simulink model "Simulacao_3DANIM"  (R2021a)
settings: Solver=ode4  StartTime=0.0  StopTime=300  FixedStep=0.01  RelTol=1e-3  EnableMultiTasking=on
values from neighbouring files (symbols this model uses):
  Ka = 4.5    [INICIO.m]
  Kdc = 1.1    [INICIO.m]
  Ki = 14.3    [INICIO.m]
  Kr = -0.37    [INICIO.m]
  l_M0 = 80*d2r    (= 1.3962634016)    [INICIO.m]
  l_T0 = -2.5*d2r    (= -0.0436332312999)    [INICIO.m]
  V_T = 600    [INICIO.m]
  X_M0 = 2000    [INICIO.m]
  X_T0 = 100    [INICIO.m]
  Z_M0 = 0    [INICIO.m]
  Z_T0 = 20000    [INICIO.m]
libraries: vrlib x3, simulink x1
settings Model: Creator=vinay  LastModifiedBy=Pedro Rocha
settings SolverCC: AlgebraicLoopSolver=TrustRegion
settings DataIOCC: LimitDataPoints=on  SaveFormat=Array  ReturnWorkspaceOutputs=off
settings OptimizationCC: LifeSpan=inf
settings DebuggingCC: SFUnexpectedBacktrackingDiag=warning  SFNoUnconditionalDefaultTransitionDiag=warning  SFExecutionAtInitializationDiag=none  SFMachineParentedDataDiag=warning  ArithmeticOperatorsInVariantConditions=warning
settings HardwareCC: ProdBitPerPointer=32  ProdBitPerSizeT=32  ProdBitPerPtrDiffT=32  ProdLargestAtomicFloat=None  ProdIntDivRoundTo=Undefined  ProdEndianess=Unspecified  ProdWordSize=32  ProdHWDeviceType=32-bit Generic
settings ModelReferenceCC: PropagateSignalLabelsOutOfModel=off
settings SFSimCC: SimUseLocalCustomCode=off  CustomCodeUndefinedFunction=UseInterfaceOnly
settings RTWCC: RTWUseLocalCustomCode=off
settings CodeAppCC: StateflowObjectComments=on
settings GRTTargetCC: TargetLangStandard=C89/C90 (ANSI)
settings ConfigComp: CovMetricSettings=dw  CovSaveCumulativeToWorkspaceVar=on  CovSaveSingleToWorkspaceVar=on  CovExternalEMLEnable=off

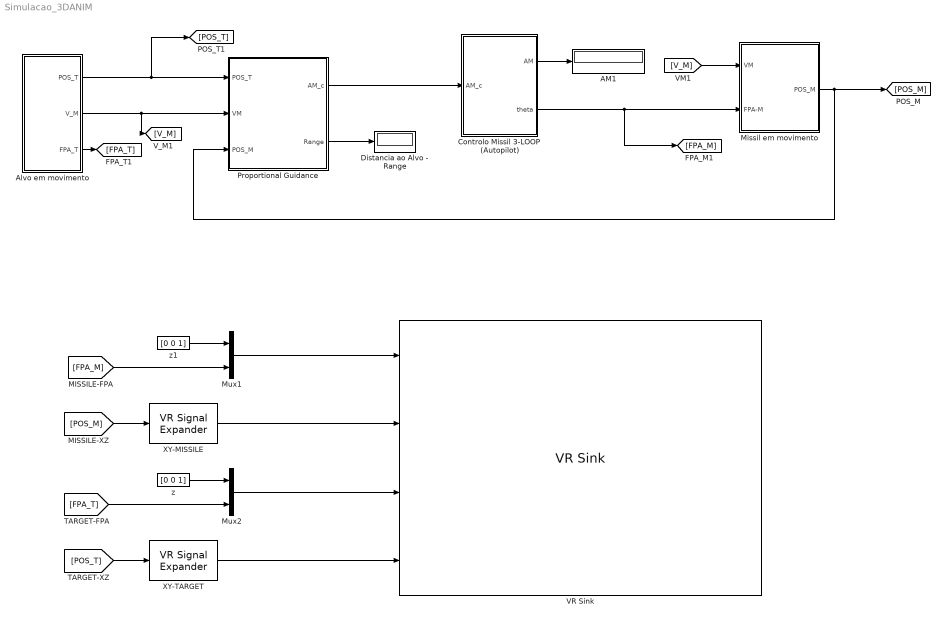
== system Simulacao_3DANIM ==
  " Controlo Missil 3-LOOP (Autopilot)" : Subsystem
  AM1 : Display
  Alvo em movimento : Subsystem
  Distancia ao Alvo - Range : Display
  Missil em movimento : Subsystem
  Mux1 : Mux  Inputs=2
  Mux2 : Mux  Inputs=2
  Proportional Guidance : Subsystem
  VR Sink : vrlib/VR Sink  InstantiateOnLoad=on  SampleTime=0.01  ViewEnable=on  RemoteChange=off  RemoteView=off  FieldsWritten=MISSILE-1_Scale.rotation.4.1.1.double#MISSILE-1_Scale.translation.3.1.1.double#UCAV_Halcyon_Test-3_Scale.rotation.4.1.1.double#UCAV_Halcyon_Test-3_Scale.translation.3.1.1.double  WorldFileName=interceptor_assembly.wrl  AutoView=off  VideoDimensions=[]  AllowVariableSize=off  FigureProperties="{'Position', 'Name', 'Viewpoint', 'CameraBound', 'CameraDirection', 'CameraPosition', 'CameraUpVector', 'ZoomFactor', 'Antialiasing', 'Headlight', 'Lighting', 'NavPanel', 'Sound', 'StatusBar', 'Stereo3D', 'Stereo3DCameraOffset', 'Stereo3DHIT', 'ToolBar', 'Textures', 'Transparency', 'Triad', 'Wireframe', 'NavZones', 'NavMode', 'NavSpeed', 'CaptureFileFormat', 'CaptureFileName', 'Record2DCompressMethod', 'Record2DCompressQuality', 'Record2D', 'Record2DFileName', 'Record2DFPS'; [0.0000000000000000e+00   8.4000000000000000e+01   1.3180000000000000e+03   9.0400000000000000e+02], '', 'target-view', 'on', [0.0000000000000000e+00   0.0000000000000000e+00  -1.0000000000000000e+00], [0.0000000000000000e+00   0.0000000000000000e+00   4.3999999999999995e-01], [0.0000000000000000e+00   1.0000000000000000e+00   0.0000000000000000e+00], [1.0000000000000000e+00], 'on', 'on', 'on', 'halfbar', 'on', 'on', 'off', [1.0000000149011612e-01], [0.0000000000000000e+00], 'on', 'on', 'on', 'none', 'off', 'off', 'walk', 'veryslow', 'tif', '%f_anim_%n.tif', 'auto', [7.5000000000000000e+01], 'off', '%f_anim_%n.avi', 'auto'}"
  XY-MISSILE : vrlib/VR Signal Expander  outwidth=3  outidx=[1 2]
  XY-TARGET : vrlib/VR Signal Expander  outwidth=3  outidx=[1 2]
  z : Constant  Value=[0 0 1]
  z1 : Constant  Value=[0 0 1]
  wires:
  [POS_T] -> XY-TARGET/1
  [POS_M] -> XY-MISSILE/1
  [FPA_M] -> Mux1/2
  [FPA_T] -> Mux2/2
  z1/1 -> Mux1/1
  z/1 -> Mux2/1
  XY-MISSILE/1 -> VR Sink/2
  Mux2/1 -> VR Sink/3
  Mux1/1 -> VR Sink/1
  XY-TARGET/1 -> VR Sink/4
  Proportional Guidance/1(AM_c) -> " Controlo Missil 3-LOOP (Autopilot)"/1(AM_c)
  [V_M] -> Missil em movimento/1(VM)
  " Controlo Missil 3-LOOP (Autopilot)"/2(theta) -> [FPA_M], Missil em movimento/2(FPA-M)
  " Controlo Missil 3-LOOP (Autopilot)"/1(AM) -> AM1/1
  Missil em movimento/1(POS_M) -> [POS_M], Proportional Guidance/3(POS_M)
  Proportional Guidance/2(Range) -> Distancia ao Alvo - Range/1
  Alvo em movimento/2(V_M) -> [V_M], Proportional Guidance/2(VM)
  Alvo em movimento/1(POS_T) -> [POS_T], Proportional Guidance/1(POS_T)
  Alvo em movimento/3(FPA_T) -> [FPA_T]

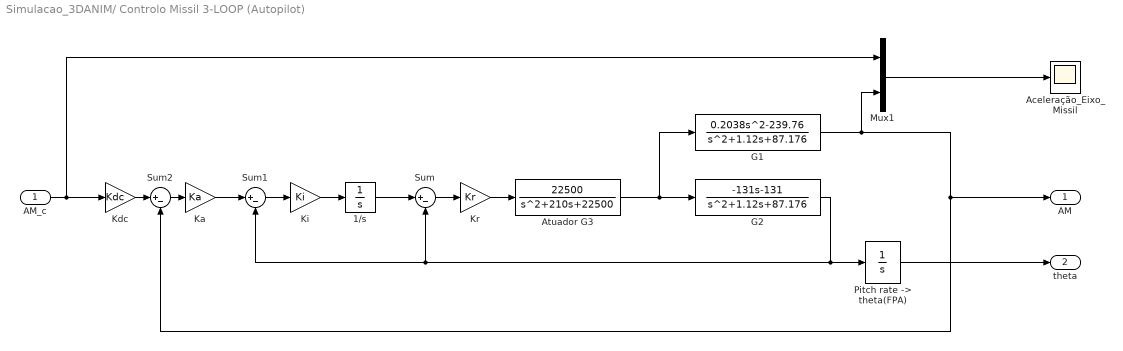
== system Simulacao_3DANIM/ Controlo Missil 3-LOOP (Autopilot) ==
  AM_c : Inport
  1/s : Integrator
  Aceleração_Eixo_Missil : Scope
  Atuador G3 : TransferFcn  Numerator=[22500]  Denominator=[1, 210, 22500]
  G1 : TransferFcn  Numerator=[0.2038, 0, -239.76]  Denominator=[1, 1.12, 87.176]
  G2 : TransferFcn  Numerator=[-131, -131]  Denominator=[1, 1.12, 87.176]
  Ka : Gain  Gain=Ka
  Kdc : Gain  Gain=Kdc
  Ki : Gain  Gain=Ki
  Kr : Gain  Gain=Kr
  Mux1 : Mux  Inputs=2
  "Pitch rate -> theta(FPA)" : Integrator  InitialCondition=l_M0
  Sum : Sum  Inputs=|+-
  Sum1 : Sum  Inputs=|+-
  Sum2 : Sum  Inputs=|+-
  AM : Outport
  theta : Outport  Port=2
  wires:
  Ki/1 -> 1/s/1
  Sum1/1 -> Ki/1
  "Pitch rate -> theta(FPA)"/1 -> theta/1
  Atuador G3/1 -> G1/1, G2/1
  Kr/1 -> Atuador G3/1
  G2/1 -> "Pitch rate -> theta(FPA)"/1, Sum/2, Sum1/2
  Sum/1 -> Kr/1
  1/s/1 -> Sum/1
  Ka/1 -> Sum1/1
  Kdc/1 -> Sum2/1
  Sum2/1 -> Ka/1
  AM_c/1 -> Kdc/1, Mux1/1
  G1/1 -> Mux1/2, AM/1, Sum2/2
  Mux1/1 -> Aceleração_Eixo_Missil/1

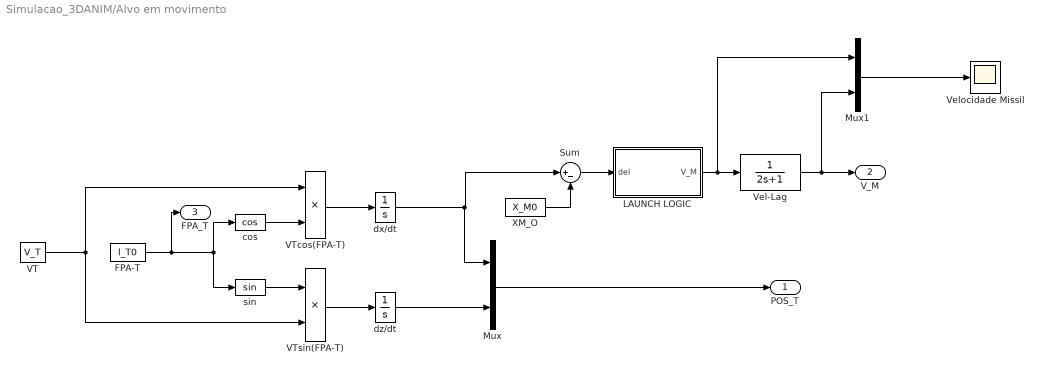
== system Simulacao_3DANIM/Alvo em movimento ==
  FPA-T : Constant  Value=l_T0
  LAUNCH LOGIC : MATLAB Function  TreatAsAtomicUnit=on
  Mux : Mux  Inputs=2
  Mux1 : Mux  Inputs=2
  Sum : Sum  Inputs=|+-
  VT : Constant  Value=V_T
  VTcos(FPA-T) : Product
  VTsin(FPA-T) : Product
  Vel-Lag : TransferFcn  Denominator=[2 1]
  Velocidade Missil : Scope
  XM_O : Constant  Value=X_M0
  cos : Trigonometry  Operator=cos
  dx/dt : Integrator  InitialCondition=X_T0
  dz/dt : Integrator  InitialCondition=Z_T0
  sin : Trigonometry
  POS_T : Outport
  V_M : Outport  Port=2
  FPA_T : Outport  Port=3
  wires:
  cos/1 -> VTcos(FPA-T)/2
  LAUNCH LOGIC/1(V_M) -> Mux1/1, Vel-Lag/1
  dx/dt/1 -> Mux/1, Sum/1
  Sum/1 -> LAUNCH LOGIC/1(del)
  XM_O/1 -> Sum/2
  dz/dt/1 -> Mux/2
  Mux/1 -> POS_T/1
  VTsin(FPA-T)/1 -> dz/dt/1
  FPA-T/1 -> FPA_T/1, sin/1, cos/1
  VT/1 -> VTsin(FPA-T)/2, VTcos(FPA-T)/1
  sin/1 -> VTsin(FPA-T)/1
  VTcos(FPA-T)/1 -> dx/dt/1
  Vel-Lag/1 -> Mux1/2, V_M/1
  Mux1/1 -> Velocidade Missil/1

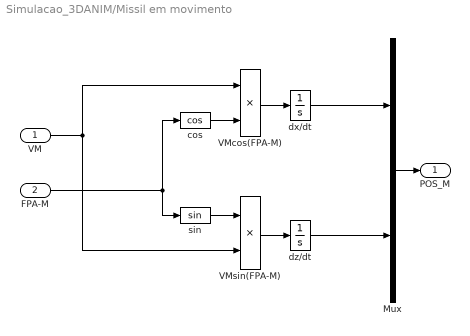
== system Simulacao_3DANIM/Missil em movimento ==
  VM : Inport
  FPA-M : Inport  Port=2
  Mux : Mux  Inputs=2
  VMcos(FPA-M) : Product
  VMsin(FPA-M) : Product
  cos : Trigonometry  Operator=cos
  dx/dt : Integrator  InitialCondition=X_M0
  dz/dt : Integrator  InitialCondition=Z_M0
  sin : Trigonometry
  POS_M : Outport
  wires:
  Mux/1 -> POS_M/1
  cos/1 -> VMcos(FPA-M)/2
  VMsin(FPA-M)/1 -> dz/dt/1
  sin/1 -> VMsin(FPA-M)/1
  VMcos(FPA-M)/1 -> dx/dt/1
  VM/1 -> VMsin(FPA-M)/2, VMcos(FPA-M)/1
  FPA-M/1 -> cos/1, sin/1
  dz/dt/1 -> Mux/2
  dx/dt/1 -> Mux/1

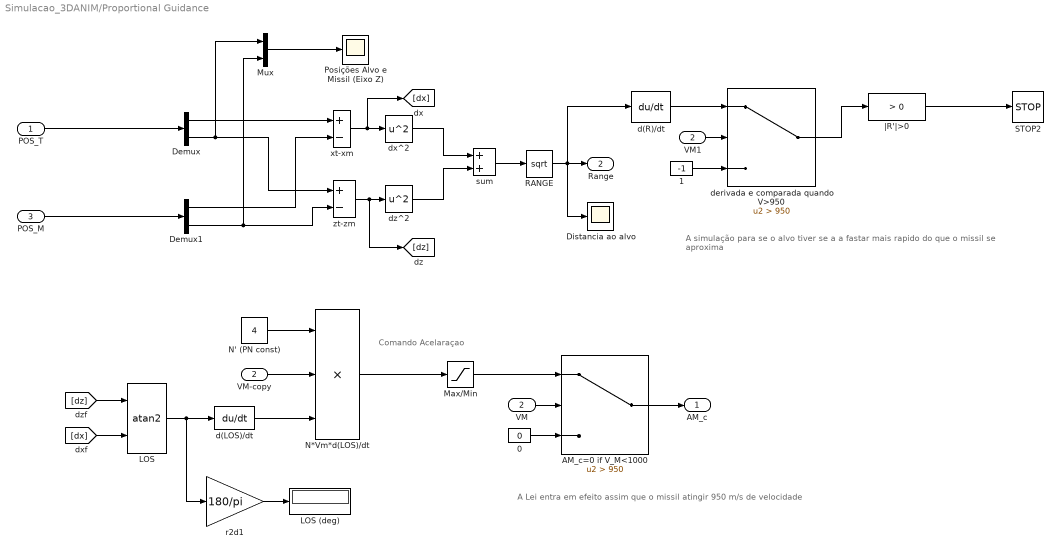
== system Simulacao_3DANIM/Proportional Guidance ==
  note: A Lei entra em efeito assim que o missil atingir 950 m/s de velocidade
  note: Comando Acelaraçao
  note: A simulação para se o alvo tiver se a a fastar mais rapido do que o missil se aproxima
  POS_T : Inport
  VM : Inport  Port=2
  POS_M : Inport  Port=3
  0 : Constant  Value=0
  1 : Constant  Value=-1
  AM_c=0 if V_M<1000 : Switch  Criteria=u2 > Threshold  Threshold=950
  Demux : Demux  Outputs=2
  Demux1 : Demux  Outputs=2
  Distancia ao alvo : Scope
  LOS : Trigonometry  Operator=atan2  OutputSignalType=real
  LOS (deg) : Display
      settings: Format=bank
  Max/Min : Saturate  UpperLimit=0.10  LowerLimit=-0.10
  Mux : Mux  Inputs=2
  N' (PN const) : Constant  Value=4
  N*Vm*d(LOS)/dt : Product  Inputs=3
  Posições Alvo e Missil (Eixo Z) : Scope
  RANGE : Sqrt  OutputSignalType=real  SaturateOnIntegerOverflow=on
  STOP2 : Stop
  VM-copy : InportShadow  Port=2
  VM1 : InportShadow  Port=2
  d(LOS)/dt : Derivative
  d(R)/dt : Derivative
  derivada e comparada quando V>950 : Switch  Criteria=u2 > Threshold  Threshold=950
  dx^2 : Math  Operator=square  SignedPower=on  OutputSignalType=real  SaturateOnIntegerOverflow=on
  dz^2 : Math  Operator=square  SignedPower=on  OutputSignalType=real  SaturateOnIntegerOverflow=on
  r2d1 : Gain  Gain=180/pi
  sum : Sum
  xt-xm : Sum  Inputs=+-
  zt-zm : Sum  Inputs=+-
  |R'|>0 : simulink/Logic and Bit Operations/Compare To Constant  relop=>  const=0  OutDataTypeStr=boolean
  AM_c : Outport
  Range : Outport  Port=2
  wires:
  AM_c=0 if V_M<1000/1 -> AM_c/1
  VM/1 -> AM_c=0 if V_M<1000/2
  POS_T/1 -> Demux/1
  POS_M/1 -> Demux1/1
  0/1 -> AM_c=0 if V_M<1000/3
  Demux/1 -> xt-xm/1
  Demux1/1 -> xt-xm/2
  Demux1/2 -> Mux/2, zt-zm/2
  Demux/2 -> Mux/1, zt-zm/1
  xt-xm/1 -> [dx], dx^2/1
  zt-zm/1 -> [dz], dz^2/1
  dx^2/1 -> sum/1
  dz^2/1 -> sum/2
  sum/1 -> RANGE/1
  RANGE/1 -> Distancia ao alvo/1, d(R)/dt/1, Range/1
  [dx] -> LOS/2
  LOS/1 -> d(LOS)/dt/1, r2d1/1
  d(LOS)/dt/1 -> N*Vm*d(LOS)/dt/3
  r2d1/1 -> LOS (deg)/1
  [dz] -> LOS/1
  N' (PN const)/1 -> N*Vm*d(LOS)/dt/1
  N*Vm*d(LOS)/dt/1 -> Max/Min/1
  VM-copy/1 -> N*Vm*d(LOS)/dt/2
  Max/Min/1 -> AM_c=0 if V_M<1000/1
  |R'|>0/1 -> STOP2/1
  Mux/1 -> Posições Alvo e Missil (Eixo Z)/1
  derivada e comparada quando V>950/1 -> |R'|>0/1
  d(R)/dt/1 -> derivada e comparada quando V>950/1
  1/1 -> derivada e comparada quando V>950/3
  VM1/1 -> derivada e comparada quando V>950/2

== matlab function Simulacao_3DANIM/Alvo em movimento/LAUNCH LOGIC ==
  settings: updateMethod=DISCRETE
  data: del input; V_M output
function V_M = fcn(del)
%#codegen

persistent f
persistent Vel

if isempty(f)
    f = 0;
end
if isempty(Vel)
    Vel = 0;
end

if f == 0 && del > -200 %missil lança quando o alvo esta a pelo menos 200 metros do missil (atras)
    f = 1;
    Vel = 1021;
end


V_M = Vel;
